simulink model "sim_Motor_2kW_closedloop_v8_delay"  (Simulink 7.9)
settings: Solver=ode45  StartTime=0.0  StopTime=0.04  RelTol=1e-3
libraries: powerlib x17, simulink_extras x1
settings Model: Creator=Kun Zhang  LastModifiedBy=LYN
settings SolverCC: AutoInsertRateTranBlk=on
settings DebuggingCC: MultiTaskDSMMsg=warning  MultiTaskCondExecSysMsg=none  StrictBusMsg=None
settings RTWCC: IncludeERTFirstTime=on
settings GRTTargetCC: CombineOutputUpdateFcns=off  GRTInterface=on

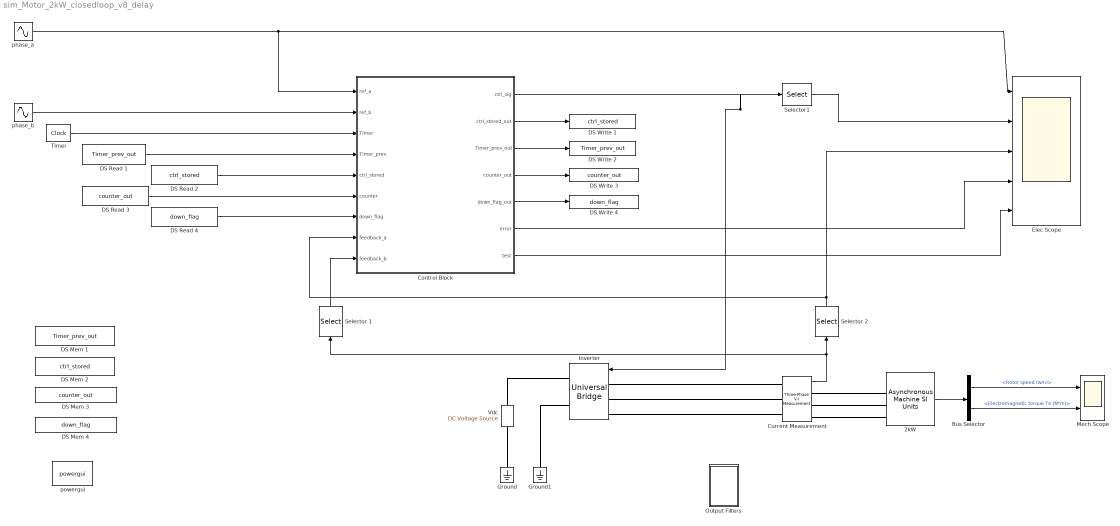
== system sim_Motor_2kW_closedloop_v8_delay ==
  2kW : powerlib/Machines/Asynchronous Machine SI Units  PresetModel=No  MechanicalLoad=Torque Tm  ShowDetailedParameters=on  RotorType=Squirrel-cage  ReferenceFrame=Rotor  NominalParameters=[ 2000, 220, 50 ]  Stator=[5 0.01]  Rotor=[ 1.083 0.005974]  Cage1=[ 0.022 0.226/377]  Cage2=[ 0.022 0.226/377]  Lm=0.2037  Mechanical=[0.02 0.005752 2]  PolePairs=2  InitialConditions=[1 0 0 0 0 0 0 0]  Units=SI  LoadFlowParameters=1492000  SimulateSaturation=off  Saturation=[14.03593122, 27.81365428, 53.79336849, 72.68890987, 97.98006896, 148.6815601, 215.7428561, 302.9841135, 428.7778367 ; 230, 322, 414, 460, 506, 552, 598, 644, 690]  TsPowergui=0  TsBlock=-1  IterativeModel=Forward Euler  Pmec=0
  Bus Selector : BusSelector  OutputSignals=Mechanical.Rotor speed (wm),Mechanical.Electromagnetic torque Te (N*m)
  Control Block : MATLAB Function  TreatAsAtomicUnit=on
  Current Measurement : powerlib/Measurements/Three-Phase V-I Measurement  VoltageMeasurement=no  SetLabelV=off  LabelV=Vabc  Vpu=off  VpuLL=off  CurrentMeasurement=yes  SetLabelI=off  LabelI=Iabc  Ipu=off  Pbase=100e6  Vbase=500e3  OutputType=Complex  PhasorSimulation=off  PSBequivalent=0
  DS Mem 1 : DataStoreMemory  DataStoreName=Timer_prev_out  ReadBeforeWriteMsg=warning  WriteAfterWriteMsg=warning  WriteAfterReadMsg=warning
  DS Mem 2 : DataStoreMemory  DataStoreName=ctrl_stored  ReadBeforeWriteMsg=warning  WriteAfterWriteMsg=warning  WriteAfterReadMsg=warning  InitialValue=[0;0;0]
  DS Mem 3 : DataStoreMemory  DataStoreName=counter_out  ReadBeforeWriteMsg=warning  WriteAfterWriteMsg=warning  WriteAfterReadMsg=warning
  DS Mem 4 : DataStoreMemory  DataStoreName=down_flag  ReadBeforeWriteMsg=warning  WriteAfterWriteMsg=warning  WriteAfterReadMsg=warning
  DS Read 1 : DataStoreRead  DataStoreName=Timer_prev_out
  DS Read 2 : DataStoreRead  DataStoreName=ctrl_stored
  DS Read 3 : DataStoreRead  DataStoreName=counter_out
  DS Read 4 : DataStoreRead  DataStoreName=down_flag
  DS Write 1 : DataStoreWrite  DataStoreName=ctrl_stored
  DS Write 2 : DataStoreWrite  DataStoreName=Timer_prev_out
  DS Write 3 : DataStoreWrite  DataStoreName=counter_out
  DS Write 4 : DataStoreWrite  DataStoreName=down_flag
  "Elec Scope " : Scope  NumInputPorts=5
      settings: TimeRange=0.00032  YMin=0.075~0~5.55112e-17~-0.1~-5  YMax=0.275~1~1~0.8~5  SaveName=motor_2kW_elec
  Ground : powerlib/Elements/Ground  LConnTagsString=a
  Ground1 : powerlib/Elements/Ground  LConnTagsString=a
  Inverter : powerlib/Power Electronics/Universal Bridge  Arms=3  SnubberResistance=5000  SnubberCapacitance=inf  Device=IGBT / Diodes  Ron=1e-3  Lon=0  ForwardVoltages="[  0  0  ]"  ForwardVoltage=0  GTOparameters=[ 10e-6 , 20e-6 ]  IGBTparameters=[ 1e-6 , 1e-6 ]  Measurements=None  Measurements_2=None  converterType=Rectifier
  Mech Scope : Scope  NumInputPorts=2
      settings: TimeRange=0.01  YMin=-1~-5  YMax=1~5  SaveName=motor_2kW_mech
  Output Filters : Subsystem
  Selector 1 : Selector  InputPortWidth=3  IndexOptions=Index vector (dialog)  Indices=[2]  OutputSizes=1
  Selector 2 : Selector  InputPortWidth=3  IndexOptions=Index vector (dialog)  Indices=[1]  OutputSizes=1
  Selector1 : Selector  InputPortWidth=6  IndexOptions=Index vector (dialog)  Indices=[1 2]  OutputSizes=1
  "Timer " : simulink_extras/Flip Flops/Clock  period=1/(20*50*1000)
  Vdc : powerlib/Electrical Sources/DC Voltage Source  Amplitude=800  Measurements=None
  "phase_a " : Sin  Frequency=2*pi*300  SampleTime=1/(100*1000)
  "phase_b " : Sin  Frequency=2*pi*300  Phase=2*pi/3  SampleTime=1/(100*1000)
  powergui : powerlib/powergui  Priority=1  SimulationMode=Discrete  SolverType=Tustin  SampleTime=1e-6  frequency=60  SPID=off  DisableSnubberDevices=off  DisableRonSwitches=off  DisableVfSwitches=off  SwTol=0  Interpol=off  DisplayEquations=off  FunctionMessages=off  frequencyindice=50  Pbase=100e6  ErrMax=1e-4  Iterations=50  UnitsV=kV  UnitsW=MW  echomessages=off  HookPort=off  EnableUseOfTLC=off  x0status=blocks  RestoreLinks=warning  ResistiveCurrentMeasurement=off  Ylog=off  Xlog=on  ShowGrid=off  save=off  variable=ZData  structure=motor_2kW_elec  ZoomFFT=off  StartTime=0.0  cycles=1  DisplayStyle=1  fundamental=60  FreqAxis=off  MaxFrequency=1000  frequencyindicesteady=1  display=off  methode=off
  wires:
  2kW/1 -> Bus Selector/1
  Bus Selector/1 -> Mech Scope/1  "<Rotor speed (wm)>"
  Bus Selector/2 -> Mech Scope/2  "<Electromagnetic torque Te (N*m)>"
  "phase_b "/1 -> Control Block/2(ref_b)
  "phase_a "/1 -> Control Block/1(ref_a), "Elec Scope "/1
  Control Block/1(ctrl_sig) -> Inverter/1, Selector1/1
  DS Read 1/1 -> Control Block/4(Timer_prev)
  Control Block/3(Timer_prev_out) -> DS Write 2/1
  DS Read 2/1 -> Control Block/5(ctrl_stored)
  Control Block/2(ctrl_stored_out) -> DS Write 1/1
  DS Read 3/1 -> Control Block/6(counter)
  Control Block/4(counter_out) -> DS Write 3/1
  "Timer "/1 -> Control Block/3(Timer)
  Current Measurement/1 -> Selector 2/1, Selector 1/1
  Selector 2/1 -> Control Block/8(feedback_a), "Elec Scope "/3
  Selector1/1 -> "Elec Scope "/2
  Selector 1/1 -> Control Block/9(feedback_b)
  Control Block/6(error) -> "Elec Scope "/4
  DS Read 4/1 -> Control Block/7(down_flag)
  Control Block/5(down_flag_out) -> DS Write 4/1
  Control Block/7(test) -> "Elec Scope "/5
  connections:
  Ground/LConn1 -- Vdc/LConn1
  Vdc/RConn1 -- Inverter/RConn1
  Inverter/RConn2 -- Ground1/LConn1
  Inverter/LConn1 -- Current Measurement/LConn1
  Inverter/LConn2 -- Current Measurement/LConn2
  Current Measurement/RConn1 -- 2kW/LConn1
  Current Measurement/RConn2 -- 2kW/LConn2
  Current Measurement/RConn3 -- 2kW/LConn3
  Inverter/LConn3 -- Current Measurement/LConn3

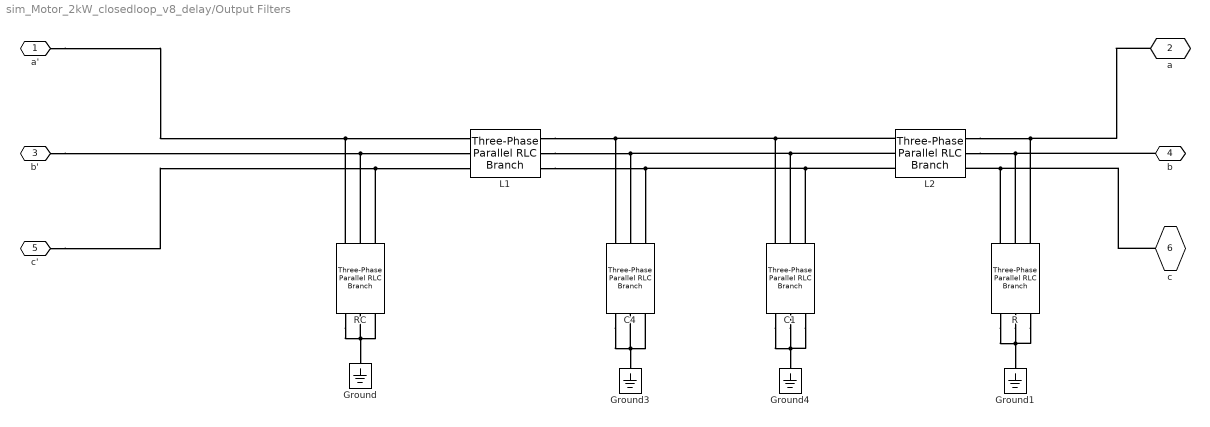
== system sim_Motor_2kW_closedloop_v8_delay/Output Filters ==
  C1 : powerlib/Elements/Three-Phase Parallel RLC Branch  LConnTagsString=A|B|C  RConnTagsString=A|B|C  BranchType=C  Resistance=1.5e6  Inductance=0.15e-5  Capacitance=10e-9  Measurements=None
  C4 : powerlib/Elements/Three-Phase Parallel RLC Branch  LConnTagsString=A|B|C  RConnTagsString=A|B|C  BranchType=C  Resistance=1.5e6  Inductance=0.15e-5  Capacitance=22e-6  Measurements=None
  Ground{,1,3..4} (4 alike) : powerlib/Elements/Ground  LConnTagsString=a
  L1 : powerlib/Elements/Three-Phase Parallel RLC Branch  LConnTagsString=A|B|C  RConnTagsString=A|B|C  BranchType=L  Resistance=1  Inductance=0.7e-1  Capacitance=1e-6  Measurements=None
  L2 : powerlib/Elements/Three-Phase Parallel RLC Branch  LConnTagsString=A|B|C  RConnTagsString=A|B|C  BranchType=L  Resistance=1  Inductance=1.4e-3  Capacitance=1e-6  Measurements=None
  "R " : powerlib/Elements/Three-Phase Parallel RLC Branch  LConnTagsString=A|B|C  RConnTagsString=A|B|C  BranchType=R  Resistance=100  Inductance=0.15e-5  Capacitance=20e-9  Measurements=None
  RC : powerlib/Elements/Three-Phase Parallel RLC Branch  LConnTagsString=A|B|C  RConnTagsString=A|B|C  BranchType=RC  Resistance=1.5e6  Inductance=0.15e-5  Capacitance=22e-6  Measurements=None
  " a'" : PMIOPort  Port=1  Side=Left
  a : PMIOPort  Port=2  Side=Right
  b' : PMIOPort  Port=3  Side=Left
  b : PMIOPort  Port=4  Side=Right
  c' : PMIOPort  Port=5  Side=Left
  c : PMIOPort  Port=6  Side=Right
  connections:
  RC/RConn1 -- " a'"/RConn1 -- L1/LConn1
  RC/RConn2 -- b'/RConn1 -- L1/LConn2
  RC/RConn3 -- c'/RConn1 -- L1/LConn3
  RC/LConn3 -- RC/LConn1 -- Ground/LConn1 -- RC/LConn2
  "R "/RConn2 -- L2/RConn2 -- b/RConn1
  "R "/LConn1 -- "R "/LConn3 -- "R "/LConn2 -- Ground1/LConn1
  L1/RConn1 -- L2/LConn1 -- C1/RConn1 -- C4/RConn1
  L1/RConn2 -- C1/RConn2 -- L2/LConn2 -- C4/RConn2
  L1/RConn3 -- C1/RConn3 -- L2/LConn3 -- C4/RConn3
  a/RConn1 -- L2/RConn1 -- "R "/RConn3
  c/RConn1 -- "R "/RConn1 -- L2/RConn3
  C4/LConn2 -- Ground3/LConn1 -- C4/LConn1 -- C4/LConn3
  C1/LConn3 -- C1/LConn1 -- Ground4/LConn1 -- C1/LConn2

== matlab function Control Block ==
  data: ref_a input double; ctrl_sig output double; ctrl_stored_out output double; ref_b input double; Timer input double; Timer_prev input double; ctrl_stored input double; Timer_prev_out output double; counter input double; down_flag input double; counter_out output double; down_flag_out output double; feedback_a input double; feedback_b input double; error output double; test output double
function [ctrl_sig,ctrl_stored_out,Timer_prev_out,counter_out,down_flag_out,error,test] = ctrl_blk_v8(ref_a,ref_b,Timer,Timer_prev,ctrl_stored,counter,down_flag,feedback_a,feedback_b)
%%%%%%%%%%%%%%%%%%%%%%%%%%%%%%%%%%%%%%%%%%%%%%%%%%%%%%%%%%%%%%%%%%%%%%%%%%%%%%%%%%%%%%%%%%%%%%%%%%%%%%%%%%%%%%%%%%%%%%%%%%%%%%%%%%%%%%%%%%%%%%%%%%%%%%%%%%%%%%%%%
%                                                                                                                                                               %
%           The aim is to:                                                                                                                                      %                                                           
%           generate 3-phase PWM waveform using principle of PWM in simulink                                                                                    %                      
%           Version 8, written by Kun Zhang                                                                                                                     %                                          
%                                                                                                                                                               %
%           The input parameters are                                                                                                                            %                                               
%           ref_a: reference signal a                                                                                                                           %                              
%           ref_b: reference signal b                                                                                                                           %         
%           t: running time                                                                                                                                     %                      
%           ton: on period                                                                                                                                      %
%           tstart: start time                                                                                                                                  %
%                                                                                                                                                               %
%%%%%%%%%%%%%%%%%%%%%%%%%%%%%%%%%%%%%%%%%%%%%%%%%%%%%%%%%%%%%%%%%%%%%%%%%%%%%%%%%%%%%%%%%%%%%%%%%%%%%%%%%%%%%%%%%%%%%%%%%%%%%%%%%%%%%%%%%%%%%%%%%%%%%%%%%%%%%%%%%
%space reserved for gloabal variables declaration

%%%%%%%%%%%%%%%%%%%%%%%%%%%%%%%%%%%%%%%%%%%%%%%%%%%%%%%%%%%%%%%%%%%%%%%%%%%%%%%%%%%%%%%%%%%%%%%%%%%%%%%%%%%%%%%%%%%%%%%%%%%%%%%%%%%%%%%%%%%%%%%%%%%%%%%%%%%%%%%%%
REF_AMP= 1;                                                                %magnitude of reference
DEAD_TIME= 1;                                                              %dead time 
Count_Max= 50;                                                             %Max counter value (50 counts= 1/20k s)
feedback_c= -feedback_a-feedback_b;

FbGain= 1/5;
feedback_a_scaled= feedback_a*FbGain;                                      %rescaling feedbacks
feedback_b_scaled= feedback_b*FbGain;
feedback_c_scaled= feedback_c*FbGain;
ref_c= -ref_a-ref_b;                                             

PropGain= 10;                                                              %proportional controller gain
%%%%%%%%%%%%%%%%%%%%%%%%%%%%%%%%%%%%%%%%%%%%%%%%%%%%%%%%%%%%%%%%%%%%%%%%%%%%%%%%%%%%%%%%%%%%%%%%%%%%%%%%%%%%%%%%%%%%%%%%%%%%%%%%%%%%%%%%%%%%%%%%%%%%%%%%%%%%%%%%%
if      counter==Count_Max                                                 %if positive edge for Timer1
                feedback_a_scaled= feedback_a*FbGain;                      %rescaling feedbacks
                feedback_b_scaled= feedback_b*FbGain;
                feedback_c_scaled= feedback_c*FbGain;
                ref_c= -ref_a-ref_b; 
                ctrl_a= (ref_a-feedback_a_scaled)*PropGain;                %control signals
                ctrl_b= (ref_b-feedback_b_scaled)*PropGain;
                ctrl_c= (ref_c-feedback_c_scaled)*PropGain;
                ctrl_a= round((ctrl_a+REF_AMP)*Count_Max/(2*REF_AMP));     %shift and scale phase a so that it ranges from 0 to 100 and digitalize
                ctrl_b= round((ctrl_b+REF_AMP)*Count_Max/(2*REF_AMP));
                ctrl_c= round((ctrl_c+REF_AMP)*Count_Max/(2*REF_AMP));  
                ctrl_stored_out= floor([ctrl_a;ctrl_b;ctrl_c]);
                down_flag= 1;
elseif  counter==0
                feedback_a_scaled= feedback_a*FbGain;                      %rescaling feedbacks
                feedback_b_scaled= feedback_b*FbGain;
                feedback_c_scaled= feedback_c*FbGain;
                ref_c= -ref_a-ref_b; 
                ctrl_a= (ref_a-feedback_a_scaled)*PropGain;                %control signals
                ctrl_b= (ref_b-feedback_b_scaled)*PropGain;
                ctrl_c= (ref_c-feedback_c_scaled)*PropGain;
                ctrl_a= round((ctrl_a+REF_AMP)*Count_Max/(2*REF_AMP));     %shift and scale phase a so that it ranges from 0 to 100 and digitalize
                ctrl_b= round((ctrl_b+REF_AMP)*Count_Max/(2*REF_AMP));
                ctrl_c= round((ctrl_c+REF_AMP)*Count_Max/(2*REF_AMP));  
                ctrl_stored_out= floor([ctrl_a;ctrl_b;ctrl_c]);
                down_flag= 0;
else
                ctrl_stored_out=  ctrl_stored;
                down_flag= down_flag;
end

%leg 1
if      counter<ctrl_stored(1)                                             %if counter is less or equal to stored phase
                pwm_1= 1;               pwm_2= 0;        
elseif  counter<ctrl_stored(1)+DEAD_TIME                                   %if counter is equal or greater than stored phase but the difference is less than dead time
                pwm_1= 0;               pwm_2= 0;
else
                pwm_1= 0;               pwm_2= 1;                           
end

%leg 2       
if      counter<ctrl_stored(2)                                         
                pwm_3= 1;               pwm_4= 0;        
elseif  counter<ctrl_stored(2)+DEAD_TIME
                pwm_3= 0;               pwm_4= 0;
else
                pwm_3= 0;               pwm_4= 1;
end

%leg 3       
if      counter<ctrl_stored(3)                                     
                pwm_5= 1;               pwm_6= 0;        
elseif  counter<ctrl_stored(3)+DEAD_TIME
                pwm_5= 0;               pwm_6= 0;
else
                pwm_5= 0;               pwm_6= 1;
end

% if      counter<DEAD_TIME                                                  %initially, pwm 1->0, delay for 5 ticks (at the rate of Timer2)                                                     
%                 pwm_1= 0;               pwm_2= 0;
%                 pwm_3= 0;               pwm_4= 0;                
%                 pwm_5= 0;               pwm_6= 0;                
% end

%if      Timer_prev<0.2 && Timer>0.8                                       %if positive edge of Timer2
if      down_flag==1
                counter= counter-1;                                        %counter ranging from 0 to 100
else  
                counter= counter+1;
end
%end

%%%%%%%%%%%%%%%%%%%%%%%%%%%%%%%%%%%%%%%%%%%%%%%%%%%%%%%%%%%%%%%%%%%%%%%%%%%%%%%%%%%%%%%%%%%%%%%%%%%%%%%%%%%%%%%%%%%%%%%%%%%%%%%%%%%%%%%%%%%%%%%%%%%%%%%%%%%%%%%%%
ctrl_sig= [pwm_1 pwm_2 pwm_3 pwm_4 pwm_5 pwm_6]';                          %six phase PWM
Timer_prev_out= Timer;
counter_out= counter;
down_flag_out= down_flag;
error= feedback_a-ref_a;
test= counter;
% plot(motor_2kW_elec.signals(1,1).values*5,'r');hold on; plot(motor_2kW_elec.signals(1,3).values);
